simulink subsystem "Shrimple_6dof_parachute_inflation"  (R2024a)
settings: Solver=VariableStepAuto  StartTime=0.0  StopTime=10.0  RelTol=1e-3
model mask{Rocket=0, Aerotable=0, main_deployment_type=ParachuteDeploymentType.Elevation_Deployment, drogue_deployment_type=ParachuteDeploymentType.Apogee_Delay_Deployment}
  mask prompts: main_deployment_type "Main Parachute Deployment"; drogue_deployment_type "Drogue Parachute Deployment"
undefined symbols (not defined in the file): Apogee_stop, Burnout_stop, COM_table, I, ignition_delay, launch_elevation, MOI_table
libraries: sharedtransform x2
settings Model: Creator=thatf  LastModifiedBy=thatf
settings RTWCC: GPUComputeCapability=3.5

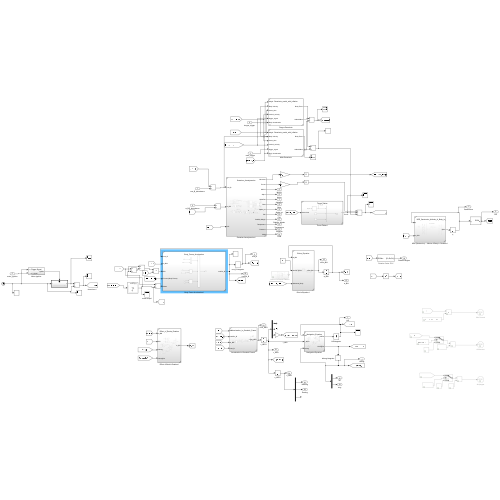
[thumbnail: Simulink's stored preview of the top-level diagram]
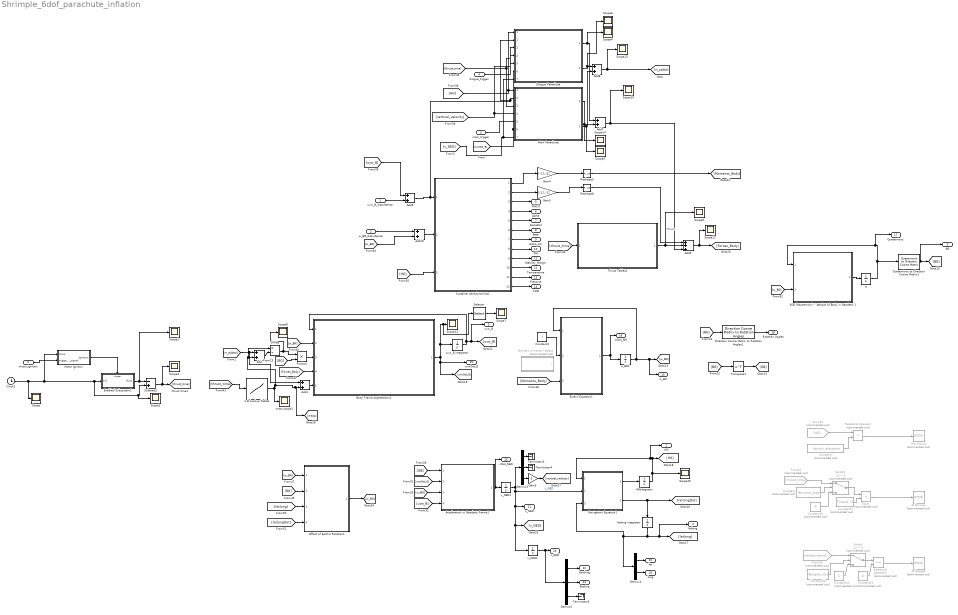
== system Shrimple_6dof_parachute_inflation ==
  uvw_B_disturbance : Inport
  w_BG_disturbance : Inport  Port=2
  main_trigger : Inport  Port=3
  drogue_trigger : Inport  Port=4
  motor_ignition : Inport  Port=5
  1-D Lookup Table1 : Lookup_n-D  NumberOfTableDimensions=1  BreakpointsForDimension1=Rocket.m_table(:,1)  Table=Rocket.m_table(:,2)  InternalRulePriority=Speed  RndMeth=Simplest
  Acceleration in Geodetic Frame1 : Subsystem  ReferencedSubsystem=Acceleration_in_Geodetic_Frame
  Add{,1,7..10} (6 alike) : Sum
  Add5 : Sum  Inputs=+++
  At Apogee : Stop  Commented=on
  At Burnout : Stop  Commented=on
  Body Frame Acceleration1 : Subsystem  ReferencedSubsystem=Body_Frame_Acceleration
  Clock2 : Clock
  Constant : Constant  Commented=on  Value=Burnout_stop
  Constant11 : Constant  Commented=on  Value=0
  Constant12 : Constant  Commented=on
  Constant13 : Constant  Commented=on  Value=Apogee_stop
  Constant16 : Constant  Commented=on  Value=0
  Constant17 : Constant  Commented=on  Value=Tx(end, 1)
  Constant2 : Constant  Value=I
  Constant7 : Constant  Commented=on  Value=launch_elevation
  Demux3 : Demux  Outputs=3
  Demux4 : Demux  Outputs=2
  Demux5 : Demux  Outputs=3
  Direction Cosine Matrix to Rotation Angles1 : sharedtransform/Direction Cosine Matrix to Rotation Angles  rotationOrder=ZYX  aMode=aMode  action=None  tolerance=eps(2)
  Divide : Product  Inputs=*/
  Drogue Parachute : Subsystem  ReferencedSubsystem=Parachute_model_with_inflation  radius=Rocket.drogue_parachute.radius  Cd=Rocket.drogue_parachute.CD  parachute_deployment_type=drogue_deployment_type  burnout_delay=0  deploy_height=Rocket.drogue_parachute.deploy_height  m_p=0.5  m_b=Rocket.m_table(end,2) - 0.5  kappa=1e7  L_SL=3
  Effect of Earth's Rotation1 : Subsystem  ReferencedSubsystem=Effect_of_Earths_Rotation
  Enabled Subsystem1 : Subsystem  TreatAsAtomicUnit=on
  Equal : RelationalOperator  Commented=on  Operator=>  OutDataTypeStr=boolean  RndMeth=Simplest  InputSameDT=off
  Euler's Equation1 : Subsystem  ReferencedSubsystem=Eulers_Equation
  From25 : From  Commented=on  GotoTag=HG
  From34 : From  Commented=on  GotoTag=vertical_velocity
  From43 : From  Commented=on  GotoTag=thrust_time
  Gain3 : Gain  Gain=-1
  Gain4 : Gain  Gain=[-1,1,-1]
  Gain5 : Gain  Gain=[-1,1,-1]
  HGIntegrator : Integrator  ContinuousStateAttributes='HG'
  Hits Ground : Stop  Commented=on
  KDE (Qauternion) -  Attidue of Body in Geodetic 1 : Subsystem  ReferencedSubsystem=KDE_Qauternion_Attitude_of_Body_in_Geodetic
  Main Parachute : Subsystem  TreatAsAtomicUnit=on  ReferencedSubsystem=Parachute_model_with_inflation  radius=Rocket.main_parachute.radius  Cd=Rocket.main_parachute.CD  parachute_deployment_type=main_deployment_type  burnout_delay=0  deploy_height=Rocket.main_parachute.deploy_height  m_p=0.8  m_b=Rocket.m_table(end,2) - 0.8  kappa=1e7  L_SL=3
      settings: MinAlgLoopOccurrences=on
  Moment of Inertia Tables1 : Subsystem  Commented=on
  Motor Ignition : Subsystem  Variant=on
  Navigation Equation1 : Subsystem  ReferencedSubsystem=Navigation_Equation
  Product : Product
  Quaternions to Direction Cosine Matrix1 : sharedtransform/Quaternions to  Direction Cosine Matrix  aMode=aMode
  Relational Operator : RelationalOperator  Commented=on  Operator=<  OutDataTypeStr=boolean  RndMeth=Simplest  InputSameDT=off
  Relational Operator1 : RelationalOperator  Commented=on  Operator=<=  OutDataTypeStr=boolean  RndMeth=Simplest  InputSameDT=off
  Reshape5 : Reshape  OutputDimensionality=Customize  OutputDimensions=[3,1]
  Reshape8 : Reshape  OutputDimensionality=Customize  OutputDimensions=[3,1]
  Scope{,1..15} (16 alike) : Scope
  Selector : Selector  InputPortWidth=3  IndexOptions=Index vector (dialog)  Indices=[1]  OutputSizes=1
  Subtract2 : Sum  Inputs=-+
  Sustainer Aerodynamics1 : Subsystem  ReferencedSubsystem=Sustainer_Aerodynamics
  Switch : Switch  Commented=on  Criteria=u2 > Threshold  SaturateOnIntegerOverflow=off  InputSameDT=off
  Switch1 : Switch  Commented=on  Criteria=u2 > Threshold  SaturateOnIntegerOverflow=off  InputSameDT=off
  Terminator3 : Terminator
  Terminator4 : Terminator
  Terminator5 : Terminator
  Thrust Tables1 : Subsystem  ReferencedSubsystem=Thrust_Tables
  Transpose1 : Math  Operator=transpose
  latlong integrator : Integrator  ContinuousStateAttributes='latlong'
  mass scope1 : Scope
  q : Integrator  ContinuousStateAttributes='q'
  uvw_B integrator : Integrator  ContinuousStateAttributes='uvw_B'
  v_NED1 : Integrator  ContinuousStateAttributes='v_NED'
  w_BN1 : Integrator  ContinuousStateAttributes='w_BN'
  x_NED1 : Integrator  ContinuousStateAttributes='position'
  HG : Outport
  BG : Outport  Port=2
  uvw_B : Outport  Port=3
  latlong : Outport  Port=4
  MACH : Outport  Port=5
  Alpha : Outport  Port=6
  AlphaDot : Outport  Port=7
  Beta : Outport  Port=8
  Alpha_tot : Outport  Port=9
  PHI : Outport  Port=10
  Stability_Margin : Outport  Port=11
  Temperature : Outport  Port=12
  Pressure : Outport  Port=13
  COM : Outport  Port=14
  w_BN : Outport  Port=15
  wDot_BN : Outport  Port=16
  Quaternions : Outport  Port=17
  Rotation Angles : Outport  Port=18
  long : Outport  Port=19
  lat : Outport  Port=20
  v_NED : Outport  Port=21
  Northing : Outport  Port=22
  Easting : Outport  Port=23
  x_NED : Outport  Port=24
  uvwDot_B : Outport  Port=25
  vDot_NED : Outport  Port=26
  wires:
  w_BG_disturbance/1 -> Add10/1
  main_trigger/1 -> Main Parachute/5
  drogue_trigger/1 -> Drogue Parachute/5
  Clock2/1 -> Enabled Subsystem1/1(In1), Subtract2/2, Scope2/1, Motor Ignition/1(time), Scope/1
  [w_BG] -> Add10/2
  Constant7/1 -> Relational Operator/2
  Motor Ignition/1(ignition) -> Enabled Subsystem1/Trigger
  Demux3/2 -> Terminator4/1
  Constant/1 -> Switch1/2
  [uvwDot_B] -> Acceleration in Geodetic Frame1/2
  Constant17/1 -> Equal/2
  HGIntegrator/1 -> [HG], HG/1, Navigation Equation1/1, Scope15/1
  Add9/1 -> Sustainer Aerodynamics1/1, Drogue Parachute/2, Main Parachute/2
  [uvw_B] -> Add9/1
  [Forces_Body] -> Body Frame Acceleration1/4
  [HG] -> Sustainer Aerodynamics1/3
  Constant12/1 -> Switch/3
  Switch1/1 -> Equal/1
  Relational Operator/1 -> Hits Ground/1
  [thrust_time] -> Main Parachute/3, Drogue Parachute/3
  Gain3/1 -> [vertical_velocity]
  Demux5/3 -> Terminator5/1
  latlong integrator/1 -> Navigation Equation1/3, Demux4/1, [latlong], latlong/1
  KDE (Qauternion) -  Attidue of Body in Geodetic 1/1 -> q/1
  [vertical_velocity] -> Main Parachute/4, Drogue Parachute/4
  Reshape5/1 -> [Moments_Body]
  Gain5/1 -> Reshape8/1
  Demux3/1 -> Terminator3/1
  Navigation Equation1/1 -> HGIntegrator/1
  Reshape8/1 -> Add5/1
  Switch/1 -> Relational Operator1/1
  x_NED1/1 -> Demux5/1, x_NED/1
  Sustainer Aerodynamics1/2 -> Gain5/1
  [BG] -> Direction Cosine Matrix to Rotation Angles1/1
  [Moments_Body] -> Euler's Equation1/3
  [HG] -> Drogue Parachute/1, Main Parachute/1
  Acceleration in Geodetic Frame1/1 -> v_NED1/1, vDot_NED/1
  Constant2/1 -> Euler's Equation1/2
  motor_ignition/1 -> Motor Ignition/2(trigger_signal)
  Navigation Equation1/2 -> latlong integrator/1, [latlongDot]
  w_BN1/1 -> Euler's Equation1/1, [w_BN], w_BN/1
  [BG] -> Effect of Earth's Rotation1/2
  q/1 -> Quaternions to Direction Cosine Matrix1/1, KDE (Qauternion) -  Attidue of Body in Geodetic 1/1, Quaternions/1
  Enabled Subsystem1/1(Out1) -> Subtract2/1, Scope1/1
  [latlongDot] -> Effect of Earth's Rotation1/4
  Effect of Earth's Rotation1/1 -> [w_BG]
  Add10/1 -> Sustainer Aerodynamics1/2
  [thrust_time] -> 1-D Lookup Table1/1
  [w_BN] -> Body Frame Acceleration1/2
  Transpose1/1 -> [GB]
  uvw_B_disturbance/1 -> Add9/2
  uvw_B integrator/1 -> Body Frame Acceleration1/1, [uvw_B], uvw_B/1
  Thrust Tables1/1 -> Add5/2, Scope9/1  "Thrust"
  Subtract2/1 -> [thrust_time], Scope3/1
  Constant11/1 -> Relational Operator1/2
  Sustainer Aerodynamics1/1 -> Gain4/1
  Euler's Equation1/1 -> w_BN1/1, wDot_BN/1
  Quaternions to Direction Cosine Matrix1/1 -> [BG], BG/1
  v_NED1/1 -> Demux3/1, [v_NED], x_NED1/1, v_NED/1, Navigation Equation1/2  "v_NED"
  Add5/1 -> [Forces_Body], Scope12/1
  From34/1 -> Switch/1
  [uvw_B] -> Acceleration in Geodetic Frame1/4
  [BG] -> Transpose1/1
  Constant13/1 -> Switch/2
  [w_BN] -> Effect of Earth's Rotation1/1
  [latlong] -> Effect of Earth's Rotation1/3
  [thrust_time] -> Thrust Tables1/1
  Sustainer Aerodynamics1/9 -> Stability_Margin/1
  Demux5/2 -> Easting/1
  Sustainer Aerodynamics1/4 -> Alpha/1
  Equal/1 -> At Burnout/1
  Constant16/1 -> Switch1/3
  Sustainer Aerodynamics1/5 -> AlphaDot/1
  Sustainer Aerodynamics1/10 -> Temperature/1
  Demux4/2 -> long/1
  Sustainer Aerodynamics1/8 -> PHI/1
  Sustainer Aerodynamics1/12 -> COM/1
  Demux3/3 -> Gain3/1
  Sustainer Aerodynamics1/6 -> Beta/1
  Sustainer Aerodynamics1/3 -> MACH/1
  [w_BG] -> KDE (Qauternion) -  Attidue of Body in Geodetic 1/2
  Demux4/1 -> lat/1
  [w_BG] -> Acceleration in Geodetic Frame1/3
  Direction Cosine Matrix to Rotation Angles1/1 -> Rotation Angles/1
  Demux5/1 -> Northing/1
  Relational Operator1/1 -> At Apogee/1
  From43/1 -> Switch1/1
  [GB] -> Acceleration in Geodetic Frame1/1
  From25/1 -> Relational Operator/1
  Gain4/1 -> Reshape5/1
  Sustainer Aerodynamics1/7 -> Alpha_tot/1
  Sustainer Aerodynamics1/11 -> Pressure/1
  Drogue Parachute/2 -> Add8/1, Scope6/1
  Main Parachute/2 -> Add8/2, Scope5/1
  Main Parachute/1 -> Scope14/1, Add7/2
  Drogue Parachute/1 -> Add7/1, Scope4/1
  1-D Lookup Table1/1 -> Divide/1, Add/2, [mass], Add1/2, mass scope1/1
  Add/1 -> Divide/2
  [BG] -> Product/2
  Product/1 -> Body Frame Acceleration1/3
  Add1/1 -> Body Frame Acceleration1/5
  [uvwDot_B] -> Drogue Parachute/6, Main Parachute/6
  Body Frame Acceleration1/1 -> uvw_B integrator/1, Scope11/1, Selector/1, uvwDot_B/1, [uvwDot_B]
  Selector/1 -> Scope7/1
  Divide/1 -> Scope8/1, Product/1
  [m_added] -> Add/1, Add1/1
  Add8/1 -> Scope13/1, [m_added]
  Add7/1 -> Scope10/1, Add5/3
  [v_NED] -> Drogue Parachute/7, Main Parachute/7

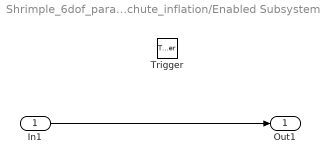
== system Shrimple_6dof_parachute_inflation/Enabled Subsystem1 ==
  In1 : Inport
  Trigger : TriggerPort  VariantControl=(inherit)  InitialTriggerSignalState=zero  PortDimensions=1
  Out1 : Outport
  wires:
  In1/1 -> Out1/1

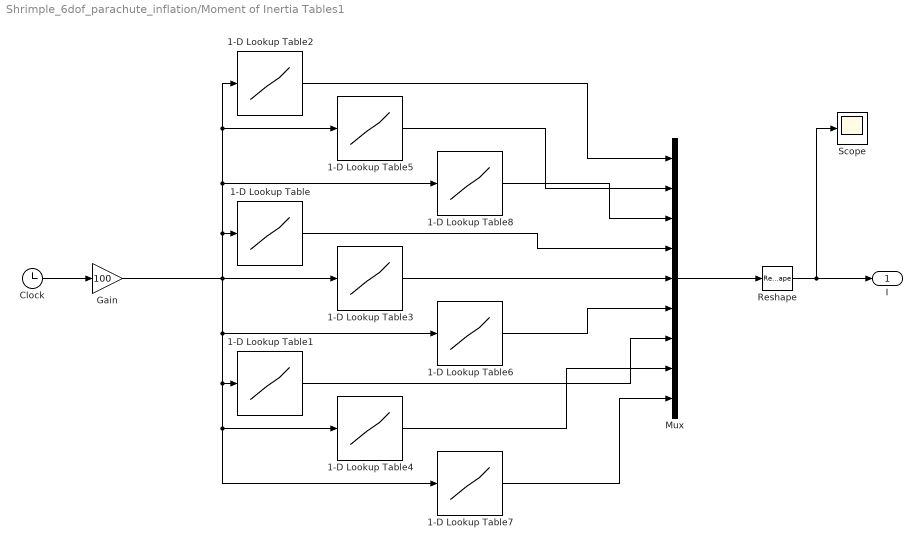
== system Shrimple_6dof_parachute_inflation/Moment of Inertia Tables1 ==
  1-D Lookup Table : Lookup_n-D  NumberOfTableDimensions=1  BreakpointsForDimension1=COM_table(:,1)  Table=MOI_table(:,2,1)  InternalRulePriority=Speed  RndMeth=Simplest
  1-D Lookup Table1 : Lookup_n-D  NumberOfTableDimensions=1  BreakpointsForDimension1=COM_table(:,1)  Table=MOI_table(:,3,1)  InternalRulePriority=Speed  RndMeth=Simplest
  1-D Lookup Table2 : Lookup_n-D  NumberOfTableDimensions=1  BreakpointsForDimension1=COM_table(:,1)  Table=MOI_table(:,1,1)  InternalRulePriority=Speed  RndMeth=Simplest
  1-D Lookup Table3 : Lookup_n-D  NumberOfTableDimensions=1  BreakpointsForDimension1=COM_table(:,1)  Table=MOI_table(:,2,2)  InternalRulePriority=Speed  RndMeth=Simplest
  1-D Lookup Table4 : Lookup_n-D  NumberOfTableDimensions=1  BreakpointsForDimension1=COM_table(:,1)  Table=MOI_table(:,3,2)  InternalRulePriority=Speed  RndMeth=Simplest
  1-D Lookup Table5 : Lookup_n-D  NumberOfTableDimensions=1  BreakpointsForDimension1=COM_table(:,1)  Table=MOI_table(:,1,2)  InternalRulePriority=Speed  RndMeth=Simplest
  1-D Lookup Table6 : Lookup_n-D  NumberOfTableDimensions=1  BreakpointsForDimension1=COM_table(:,1)  Table=MOI_table(:,2,3)  InternalRulePriority=Speed  RndMeth=Simplest
  1-D Lookup Table7 : Lookup_n-D  NumberOfTableDimensions=1  BreakpointsForDimension1=COM_table(:,1)  Table=MOI_table(:,3,3)  InternalRulePriority=Speed  RndMeth=Simplest
  1-D Lookup Table8 : Lookup_n-D  NumberOfTableDimensions=1  BreakpointsForDimension1=COM_table(:,1)  Table=MOI_table(:,1,3)  InternalRulePriority=Speed  RndMeth=Simplest
  Clock : Clock
  Gain : Gain  Gain=100
  Mux : Mux  Inputs=9
  Reshape : Reshape  OutputDimensionality=Customize  OutputDimensions=[3,3]
  Scope : Scope
  I : Outport
  wires:
  Gain/1 -> 1-D Lookup Table6/1, 1-D Lookup Table1/1, 1-D Lookup Table4/1, 1-D Lookup Table7/1, 1-D Lookup Table3/1, 1-D Lookup Table/1, 1-D Lookup Table8/1, 1-D Lookup Table5/1, 1-D Lookup Table2/1
  Reshape/1 -> I/1, Scope/1
  Mux/1 -> Reshape/1
  1-D Lookup Table7/1 -> Mux/9
  1-D Lookup Table4/1 -> Mux/8
  1-D Lookup Table1/1 -> Mux/7
  1-D Lookup Table6/1 -> Mux/6
  1-D Lookup Table3/1 -> Mux/5
  1-D Lookup Table/1 -> Mux/4
  1-D Lookup Table8/1 -> Mux/3
  1-D Lookup Table5/1 -> Mux/2
  1-D Lookup Table2/1 -> Mux/1
  Clock/1 -> Gain/1

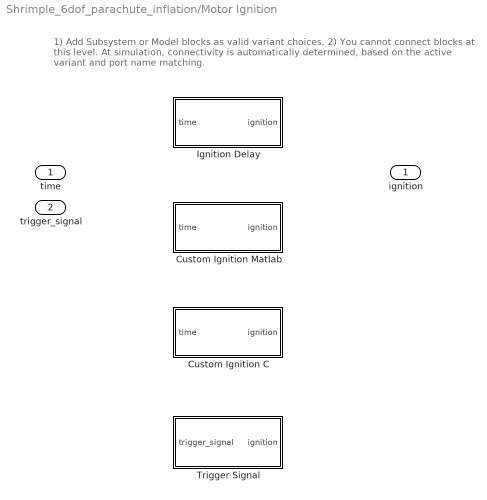
== system Shrimple_6dof_parachute_inflation/Motor Ignition ==
  note: 1) Add Subsystem or Model blocks as valid variant choices.
      | 2) You cannot connect blocks at this level. At simulation, connectivity is automatically
      | determined, based on the active variant and port name matching.
  time : Inport
  trigger_signal : Inport  Port=2
  Custom Ignition C : Subsystem  VariantControl=false
  Custom Ignition Matlab : Subsystem  VariantControl=false
  Ignition Delay : Subsystem  VariantControl=false
  Trigger Signal : Subsystem  VariantControl=true
  ignition : Outport

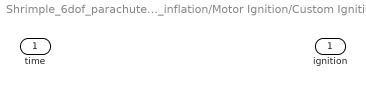
== system Shrimple_6dof_parachute_inflation/Motor Ignition/Custom Ignition C ==
  time : Inport
  ignition : Outport

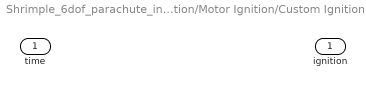
== system Shrimple_6dof_parachute_inflation/Motor Ignition/Custom Ignition Matlab ==
  time : Inport
  ignition : Outport

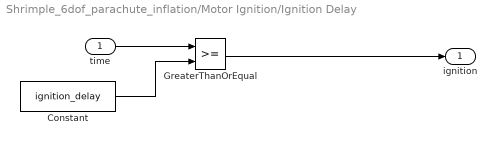
== system Shrimple_6dof_parachute_inflation/Motor Ignition/Ignition Delay ==
  time : Inport
  Constant : Constant  Value=ignition_delay
  GreaterThanOrEqual : RelationalOperator  OutDataTypeStr=boolean  RndMeth=Simplest  InputSameDT=off
  ignition : Outport
  wires:
  GreaterThanOrEqual/1 -> ignition/1
  Constant/1 -> GreaterThanOrEqual/2
  time/1 -> GreaterThanOrEqual/1

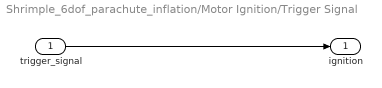
== system Shrimple_6dof_parachute_inflation/Motor Ignition/Trigger Signal ==
  trigger_signal : Inport
  ignition : Outport
  wires:
  trigger_signal/1 -> ignition/1
